simulink model "march1_2022_buckboost_conv_with_transfer_function"  (R2018a)
settings: Solver=ode45  StartTime=0.0  StopTime=0.6  RelTol=1e-3  EnableMultiTasking=on
libraries: powerlib x10
settings Model: Creator=Saman  LastModifiedBy=Faizan
settings DataIOCC: LimitDataPoints=on  SaveFormat=Array  SignalLoggingSaveFormat=ModelDataLogs
settings OptimizationCC: ExpressionDepthLimit=2147483647  LifeSpan=inf
settings DebuggingCC: UnderspecifiedInitializationDetection=Classic  MergeDetectMultiDrivingBlocksExec=none  FcnCallInpInsideContextMsg=warning  StateNameClashWarn=warning  SFUnexpectedBacktrackingDiag=warning  SFNoUnconditionalDefaultTransitionDiag=warning  SFExecutionAtInitializationDiag=none
settings HardwareCC: ProdBitPerPointer=32  ProdBitPerSizeT=32  ProdBitPerPtrDiffT=32  ProdLargestAtomicFloat=None  ProdIntDivRoundTo=Undefined  ProdEndianess=Unspecified  ProdWordSize=32  ProdHWDeviceType=32-bit Generic
settings ModelReferenceCC: PropagateSignalLabelsOutOfModel=off
settings CodeAppCC: StateflowObjectComments=on
settings GRTTargetCC: TargetLangStandard=C89/C90 (ANSI)  CombineOutputUpdateFcns=off  GRTInterface=on
settings ConfigComp: CovMetricSettings=dw  CovHtmlReporting=on  CovSaveCumulativeToWorkspaceVar=on  CovSaveSingleToWorkspaceVar=on  CovExternalEMLEnable=off

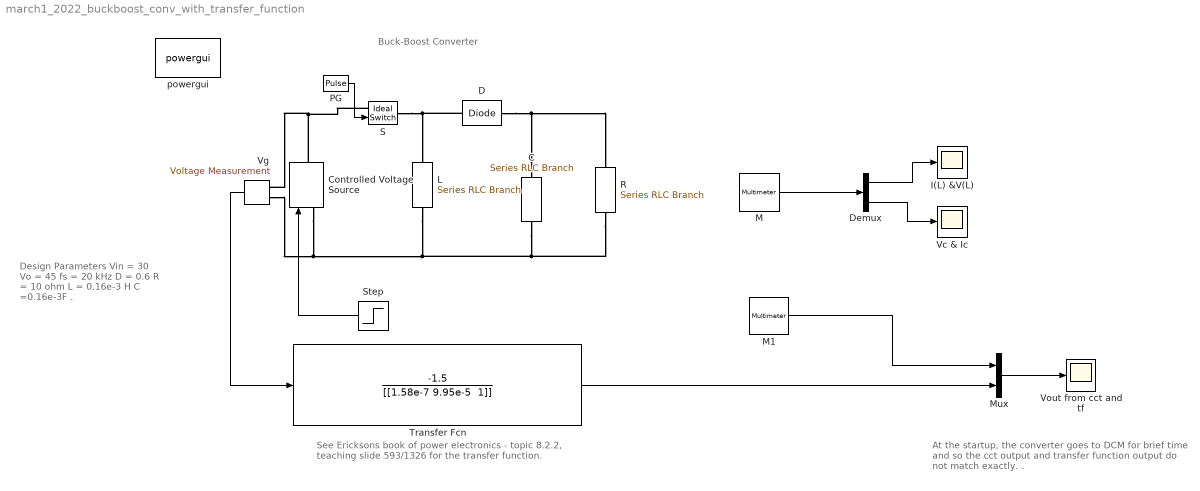
== system march1_2022_buckboost_conv_with_transfer_function ==
  note: Buck-Boost Converter
  note: Design Parameters
      |
      | Vin = 30
      | Vo = 45
      | fs = 20 kHz
      | D = 0.6
      | R = 10 ohm
      | L = 0.16e-3 H
      | C =0.16e-3F
      | .
  note: At the startup, the converter goes to DCM for
      | brief time and so the cct output and transfer function
      | output do not match exactly. .
  note: See Ericksons book of power electronics - topic 8.2.2,
      | teaching slide 593/1326 for the transfer function.
  C : powerlib/Elements/Series RLC Branch  LConnTagsString=__new0  RConnTagsString=__new0  BranchType=C  Resistance=1  Inductance=1e-3  SetiL0=off  InitialCurrent=0  Capacitance=0.16e-3  Setx0=off  InitialVoltage=0  Measurements=Branch voltage and current
  Controlled Voltage Source : powerlib/Electrical Sources/Controlled Voltage Source  Initialize=on  Source_Type=DC  Amplitude=30  Phase=0  Frequency=0  Measurements=None
  D : powerlib/Power Electronics/Diode  Ron=0.001  Lon=0  Vf=0.01  IC=0  UseSnubber=off  Rs=0  Cs=0  Measurements=off
  Demux : Demux  Outputs=2
  I(L) &V(L) : Scope
  L : powerlib/Elements/Series RLC Branch  LConnTagsString=__new0  RConnTagsString=__new0  BranchType=L  Resistance=1  Inductance=0.16e-3  SetiL0=off  InitialCurrent=0  Capacitance=1e-6  Setx0=off  InitialVoltage=0  Measurements=Branch voltage and current
  M : powerlib/Measurements/Multimeter  PhasorSimulation=off  OutputType=Complex  sel=[5 2 4 1]  L=5  Gain=[1 1 1 1]  yselected={'Ib: L','Ub: L','Ib: C','Ub: C'};  PSBOutputType=1  PSBequivalent=0  AxesSetting=[0,0.1,-100,100]  Display=0  SavedBlockNames=-11
  M1 : powerlib/Measurements/Multimeter  PhasorSimulation=off  OutputType=Complex  sel=1  L=5  Gain=1  yselected={'Ub: C'};  PSBOutputType=1  PSBequivalent=0  AxesSetting=[0,0.1,-100,100]  Display=0  SavedBlockNames=-11
  Mux : Mux  Inputs=2
  PG : DiscretePulseGenerator  PulseType=Time based  Period=5e-5  PulseWidth=60
  R : powerlib/Elements/Series RLC Branch  LConnTagsString=__new0  RConnTagsString=__new0  BranchType=R  Resistance=10  Inductance=1e-3  SetiL0=off  InitialCurrent=0  Capacitance=1e-6  Setx0=off  InitialVoltage=0  Measurements=Branch voltage
  S : powerlib/Power Electronics/Ideal Switch  Ron=0.001  Lon=0  IC=0  Rs=1e5  Cs=inf  Measurements=off
  Step : Step  Time=0.3  Before=30  After=35  SampleTime=0
  Transfer Fcn : TransferFcn  Numerator=[-1.5]  Denominator="[[1.58e-7 9.95e-5  1]]"
  Vc & Ic : Scope
  Vg : powerlib/Measurements/Voltage Measurement  PhasorSimulation=off  OutputType=Complex  PSBequivalent=0
  Vout from cct and tf : Scope
  powergui : powerlib/powergui  Priority=1  SimulationMode=Continuous  SampleTime=50e-6  frequency=60  Iterations=50  frequencyindice=0  Pbase=100e6  ErrMax=1e-4  UnitsV=kV  UnitsW=MW  buscounter=0  FunctionMessages=off  echomessages=off  EnableUseOfTLC=off  CurrentSourceSwitches=on  DisableSnubberDevices=off  DisableRonSwitches=off  DisableVfSwitches=off  DisplayEquations=off  SolverType=Tustin/Backward Euler (TBE)  Interpol=off  ExternalGateDelay=off  methode=off  Ts=0  x0status=blocks  SPID=off  SwTol=0  HookPort=off  RestoreLinks=warning  ResistiveCurrentMeasurement=off  Frange=[0:2:500]  Ylog=off  Xlog=on  ShowGrid=off  save=off  variable=ZData  structure=0  ZoomFFT=on  StartTime=0.0  cycles=1  DisplayStyle=1  fundamental=60  FreqAxis=off  MaxFrequency=1000  frequencyindicesteady=1  RmsSteady=1  display=off
  wires:
  PG/1 -> S/1
  M/1 -> Demux/1
  Demux/1 -> I(L) &V(L)/1
  Demux/2 -> Vc & Ic/1
  Vg/1 -> Transfer Fcn/1
  Transfer Fcn/1 -> Mux/2
  M1/1 -> Mux/1
  Mux/1 -> Vout from cct and tf/1
  Step/1 -> Controlled Voltage Source/1
  connections:
  C/RConn1 -- R/RConn1 -- L/RConn1 -- Controlled Voltage Source/LConn1 -- Vg/LConn2
  D/RConn1 -- S/RConn1 -- L/LConn1
  C/LConn1 -- D/LConn1 -- R/LConn1
  Controlled Voltage Source/RConn1 -- S/LConn1 -- Vg/LConn1
